simulink library "Q_solar_function"  (R2025b)
settings: Solver=VariableStepAuto  StartTime=0.0  StopTime=10.0  RelTol=1e-3
settings Model: Creator=cdt  LastModifiedBy=cdt

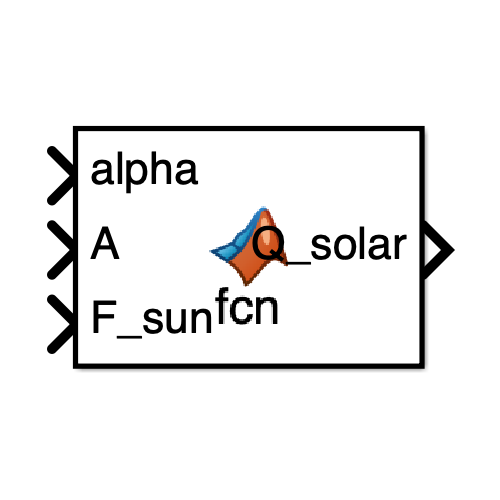
[thumbnail: Simulink's stored preview of the top-level diagram]
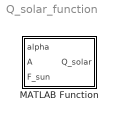
== system Q_solar_function ==
  MATLAB Function : MATLAB Function  TreatAsAtomicUnit=on

== matlab function Q_solar_function/MATLAB Function ==
  data: alpha input; Q_solar output; A input; F_sun input
function Q_solar = fcn(alpha, A, F_sun)
%Q_solar: total solvarmeeffekt (W)
%alpha: sol-absorptans af materiale (forskellig for MLI og radiator)
%A: areal af overflade (m^2)
%F_sun: solens indfaldsvinkel-faktor (cos(theta) når solen rammer, 0 i skygge)

G_s = 1361; % Solarkonstant W/m^2

Q_solar = alpha * G_s * A * F_sun;
